simulink model "neptune_IDFT_HDL_Coder_input"  (R2023a)
settings: Solver=FixedStepDiscrete  StartTime=0.0  StopTime=20*(1/20000)  RelTol=1e-3  EnableMultiTasking=on
values from neighbouring files (symbols this model uses):
  AgcBurst = fi(AgcBurst)    [ofdm.m]
  PTT = timeseries(PTT, 1/22120448)    [ofdm.m]
undefined symbols (not defined in the file or in its folder): PreambleAlong, PreambleAshort, PreambleB
libraries: hdlsllib x10, dspsigops x4, commrandsrc3 x2, dsphdlxfrm2 x2, dspstat3 x1
settings Model: Creator=abraxas3d  LastModifiedBy=matt
settings OptimizationCC: BlockReduction=off  ConditionallyExecuteInputs=off  DefaultParameterBehavior=Inlined
settings DebuggingCC: AlgebraicLoopMsg=error  SingleTaskRateTransMsg=error
settings HardwareCC: ProdBitPerPointer=32  ProdBitPerSizeT=32  ProdBitPerPtrDiffT=32  ProdLargestAtomicFloat=None  ProdIntDivRoundTo=Undefined  ProdEndianess=Unspecified  ProdWordSize=32  ProdHWDeviceType=ASIC/FPGA->ASIC/FPGA  TargetBitPerLong=64  TargetBitPerPointer=64  TargetBitPerSizeT=64  TargetBitPerPtrDiffT=64  TargetLongLongMode=on  TargetIntDivRoundTo=Zero  TargetEndianess=LittleEndian  TargetWordSize=64  TargetHWDeviceType=Custom Processor->MATLAB Host Computer  ProdEqTarget=off

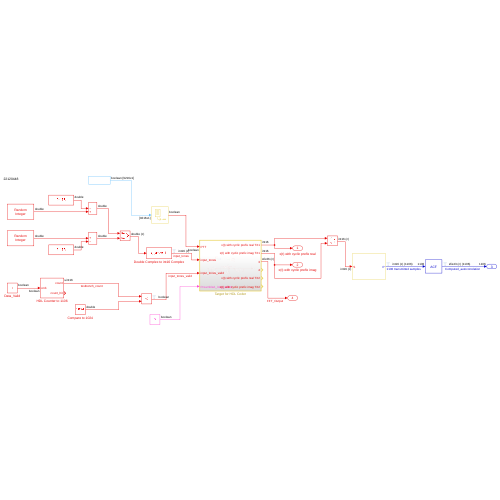
[thumbnail: Simulink's stored preview of the top-level diagram]
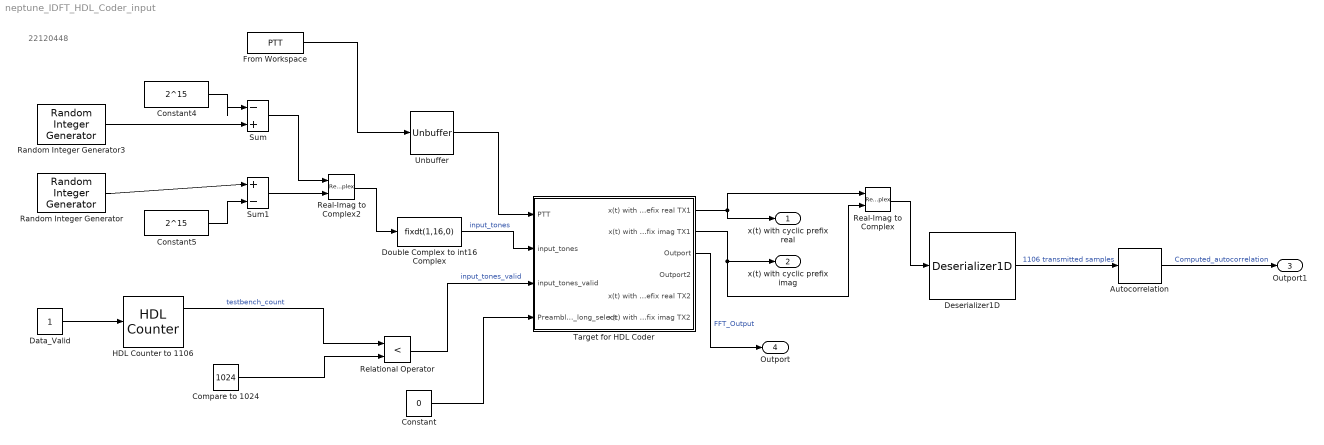
== system neptune_IDFT_HDL_Coder_input ==
  note: 22120448
  Autocorrelation : dspstat3/Autocorrelation  AllPositiveLags=on  maxlag=1105  bias=Unbiased  domain=Time  roundingMode=Floor  overflowMode=off  outputDataTypeStr=Inherit: Same as accumulator  outputMin=[]  outputMax=[]  outputLastDataTypeStr=Inherit: Same as accumulator
  Compare to 1024 : Constant  Value=1024  SampleTime=(1/22120448)
  Constant : Constant  Value=0  OutDataTypeStr=boolean
  Constant4 : Constant  Value=2^15  SampleTime=1/22120448
  Constant5 : Constant  Value=2^15  SampleTime=1/22120448
  Data_Valid : Constant  OutDataTypeStr=boolean  SampleTime=(1/22120448)
  Deserializer1D : hdlsllib/HDL Operations/Deserializer1D  Ratio=1106  IdleCycles=0  InitialCondition=0  startIn=off  validIn=off  validOut=off  inputDataDimensions=-1  inputSampleTime=-1  inputSignalType=complex
  Double Complex to int16 Complex : DataTypeConversion  OutMin=[-32768]  OutMax=[32767]  OutDataTypeStr=fixdt(1,16,0)  RndMeth=Floor
  From Workspace : FromWorkspace  VariableName=PTT  SampleTime=size(PTT.Data, 1)/22120448
  HDL Counter to 1106 : hdlsllib/Sources/HDL Counter  CountType=Count limited  CountInit=0  CountStep=1  CountMax=1105  CountFromType=Initial value  CountFrom=0  CountResetPort=off  CountLoadPort=off  CountEnbPort=on  CountDirPort=off  CountHitOutputPort=on  CountDataType=Unsigned  CountWordLen=16  CountFracLen=0  CountSampTime=1
  Random Integer Generator : commrandsrc3/Random Integer Generator  SetSize=2^16  SeedSource=Auto  Seed=0  SampleTime=1/22120448  SamplesPerFrame=1  OutputDataType=double  SimulateUsing=Interpreted execution
  Random Integer Generator3 : commrandsrc3/Random Integer Generator  SetSize=2^16  SeedSource=Auto  Seed=0  SampleTime=1/22120448  SamplesPerFrame=1  OutputDataType=double  SimulateUsing=Interpreted execution
  Real-Imag to Complex : RealImagToComplex
  Real-Imag to Complex2 : RealImagToComplex
  Relational Operator : RelationalOperator  Operator=<  OutDataTypeStr=boolean  InputSameDT=off
  Sum : Sum  Inputs=|-+
  Sum1 : Sum  Inputs=|+-
  Target for HDL Coder : Subsystem  TreatAsAtomicUnit=on
  Unbuffer : Unbuffer
  x(t) with cyclic prefix real : Outport
  x(t) with cyclic prefix imag : Outport  Port=2  VectorParamsAs1DForOutWhenUnconnected=off
  Outport1 : Outport  Port=3
  Outport : Outport  Port=4
  wires:
  Double Complex to int16 Complex/1 -> Target for HDL Coder/2(input_tones)  "input_tones"
  Target for HDL Coder/1(x(t) with cyclic prefix real TX1) -> x(t) with cyclic prefix real/1, Real-Imag to Complex/1
  Target for HDL Coder/2(x(t) with cyclic prefix imag TX1) -> Real-Imag to Complex/2, x(t) with cyclic prefix imag/1
  Compare to 1024/1 -> Relational Operator/2
  HDL Counter to 1106/1 -> Relational Operator/1  "testbench_count"
  Relational Operator/1 -> Target for HDL Coder/3(input_tones_valid)  "input_tones_valid"
  Data_Valid/1 -> HDL Counter to 1106/1
  Real-Imag to Complex/1 -> Deserializer1D/1
  Deserializer1D/1 -> Autocorrelation/1  "1106 transmitted samples"
  Autocorrelation/1 -> Outport1/1  "Computed_autocorrelation"
  Real-Imag to Complex2/1 -> Double Complex to int16 Complex/1
  Random Integer Generator3/1 -> Sum/2
  Constant4/1 -> Sum/1
  Sum/1 -> Real-Imag to Complex2/1
  Constant5/1 -> Sum1/2
  Random Integer Generator/1 -> Sum1/1
  Sum1/1 -> Real-Imag to Complex2/2
  Target for HDL Coder/3(Outport) -> Outport/1  "FFT_Output"
  Unbuffer/1 -> Target for HDL Coder/1(PTT)
  From Workspace/1 -> Unbuffer/1
  Constant/1 -> Target for HDL Coder/4(PreambleA_long_select)

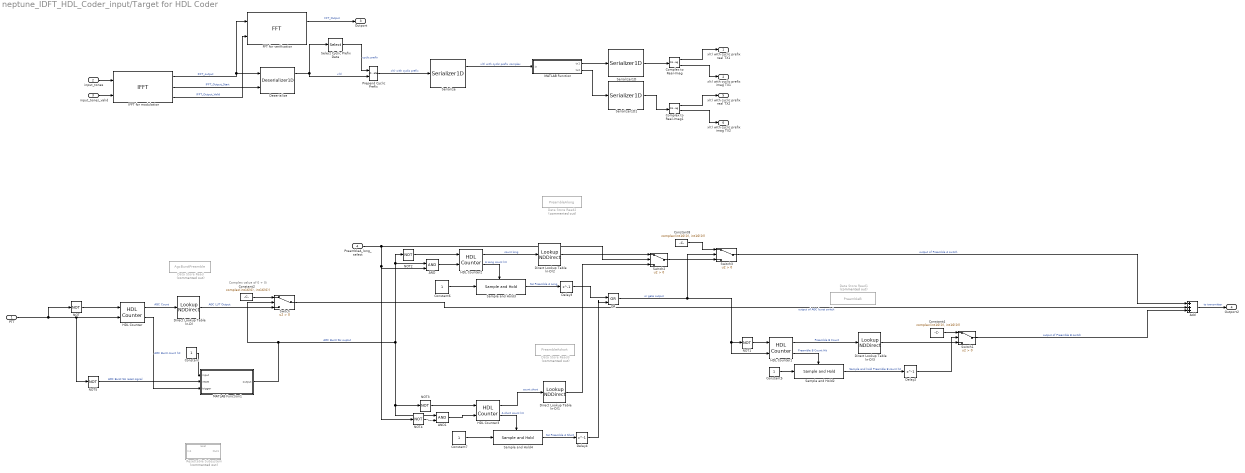
== system neptune_IDFT_HDL_Coder_input/Target for HDL Coder ==
  note: Complex value of 0 + 0i
  PTT : Inport  OutDataTypeStr=boolean
  input_tones : Inport  Port=2
  input_tones_valid : Inport  Port=3
  PreambleA_long_select : Inport  Port=4
  AND : Logic  IconShape=distinctive  AllPortsSameDT=off  OutDataTypeStr=boolean
  AND1 : Logic  IconShape=distinctive  AllPortsSameDT=off  OutDataTypeStr=boolean
  Add : Sum  Inputs=+++  OutDataTypeStr=fixdt(1,16,0)  SaturateOnIntegerOverflow=on
  Complex to Real-Imag : ComplexToRealImag
  Complex to Real-Imag1 : ComplexToRealImag
  Constant : Constant  OutDataTypeStr=boolean
  Constant2 : Constant  Value=complex(int16(0), int16(0))  VectorParams1D=off  OutDataTypeStr=int16
  Constant4 : Constant  Value=complex(int16(0), int16(0))  VectorParams1D=off  OutDataTypeStr=int16
  Constant5 : Constant  VectorParams1D=off  OutDataTypeStr=boolean  SampleTime=-1
  Constant6 : Constant  VectorParams1D=off  OutDataTypeStr=boolean  SampleTime=-1
  Constant7 : Constant  VectorParams1D=off  OutDataTypeStr=boolean  SampleTime=-1
  Constant8 : Constant  Value=complex(int16(0), int16(0))  VectorParams1D=off  OutDataTypeStr=int16
  Data Store Read : DataStoreRead  Commented=on  DataStoreName=AgcBurstPreamble  DataStoreElements=AgcBurstPreamble  EnableIndexing=on  IndexOptions=Index vector (port)  Indices=1  OutputSizes=1
  Data Store Read1 : DataStoreRead  Commented=on  DataStoreName=PreambleB  DataStoreElements=PreambleB  EnableIndexing=on  IndexOptions=Index vector (port)  Indices=1  OutputSizes=1
  Data Store Read2 : DataStoreRead  Commented=on  DataStoreName=PreambleAlong  DataStoreElements=PreambleAlong  EnableIndexing=on  IndexOptions=Index vector (port)  Indices=1  OutputSizes=1
  Data Store Read3 : DataStoreRead  Commented=on  DataStoreName=PreambleAshort  DataStoreElements=PreambleAshort  EnableIndexing=on  IndexOptions=Index vector (port)  Indices=1  OutputSizes=1
  Delay2 : Delay  DelayLength=1
  Delay3 : Delay  DelayLength=1
  Delay4 : Delay  DelayLength=1
  Deserialize : hdlsllib/HDL Operations/Deserializer1D  Ratio=1024  IdleCycles=82  InitialCondition=0  startIn=on  validIn=off  validOut=on  inputDataDimensions=-1  inputSampleTime=-1  inputSignalType=auto
  Direct Lookup Table (n-D) : LookupNDDirect  NumberOfTableDimensions=1  Table=AgcBurst  DiagnosticForOutOfRangeInput=Error
  Direct Lookup Table (n-D)1 : LookupNDDirect  NumberOfTableDimensions=1  Table=PreambleAshort  DiagnosticForOutOfRangeInput=Error
  Direct Lookup Table (n-D)2 : LookupNDDirect  NumberOfTableDimensions=1  Table=PreambleAlong  DiagnosticForOutOfRangeInput=Error
  Direct Lookup Table (n-D)3 : LookupNDDirect  NumberOfTableDimensions=1  Table=PreambleB  DiagnosticForOutOfRangeInput=Error
  FFT for verification : dsphdlxfrm2/FFT  FFTLength=1024  Architecture=Streaming Radix 2^2  ComplexMultiplication=Use 4 multipliers and 2 adders  BitReversedOutput=off  BitReversedInput=on  Normalize=off  SimulateUsing=Code generation  RoundingMethod=Floor  ResetInputPort=off  StartOutputPort=off  EndOutputPort=off
  HDL Counter : hdlsllib/Sources/HDL Counter  CountType=Count limited  CountInit=0  CountStep=1  CountMax=109  CountFromType=Initial value  CountFrom=0  CountResetPort=on  CountLoadPort=off  CountEnbPort=on  CountDirPort=off  CountHitOutputPort=on  CountDataType=Unsigned  CountWordLen=8  CountFracLen=0  CountSampTime=1
  HDL Counter1 : hdlsllib/Sources/HDL Counter  CountType=Count limited  CountInit=0  CountStep=1  CountMax=1024  CountFromType=Initial value  CountFrom=0  CountResetPort=on  CountLoadPort=off  CountEnbPort=on  CountDirPort=off  CountHitOutputPort=on  CountDataType=Unsigned  CountWordLen=16  CountFracLen=0  CountSampTime=1
  HDL Counter2 : hdlsllib/Sources/HDL Counter  CountType=Count limited  CountInit=1  CountStep=1  CountMax=5530  CountFromType=Initial value  CountFrom=1  CountResetPort=on  CountLoadPort=off  CountEnbPort=on  CountDirPort=off  CountHitOutputPort=on  CountDataType=Unsigned  CountWordLen=16  CountFracLen=0  CountSampTime=1
  HDL Counter3 : hdlsllib/Sources/HDL Counter  CountType=Count limited  CountInit=0  CountStep=1  CountMax=552  CountFromType=Initial value  CountFrom=0  CountResetPort=on  CountLoadPort=off  CountEnbPort=on  CountDirPort=off  CountHitOutputPort=on  CountDataType=Unsigned  CountWordLen=16  CountFracLen=0  CountSampTime=1
  IFFT for modulation : dsphdlxfrm2/IFFT  FFTLength=IFFTsize  Architecture=Streaming Radix 2^2  ComplexMultiplication=Use 4 multipliers and 2 adders  BitReversedOutput=on  BitReversedInput=off  Normalize=on  SimulateUsing=Code generation  RoundingMethod=Floor  ResetInputPort=off  StartOutputPort=on  EndOutputPort=off
  MATLAB Function : MATLAB Function  TreatAsAtomicUnit=on
  MATLAB Function1 : MATLAB Function  TreatAsAtomicUnit=on
  NOT{,1..5} (6 alike) : Logic  Operator=NOT  IconShape=distinctive  AllPortsSameDT=off  OutDataTypeStr=boolean
  OR : Logic  Operator=OR  IconShape=distinctive  AllPortsSameDT=off  OutDataTypeStr=boolean
  Prepend Cyclic Prefix : Concatenate
  Resettable Subsystem : Subsystem  Commented=on  TreatAsAtomicUnit=on
  Sample and Hold2 : dspsigops/Sample and Hold  trig=Rising edge  initCond=0  latchinput=off
  Sample and Hold3 : dspsigops/Sample and Hold  trig=Rising edge  initCond=0  latchinput=off
  Sample and Hold4 : dspsigops/Sample and Hold  trig=Rising edge  initCond=0  latchinput=off
  Select Cyclic Prefix Data : Selector  InputPortWidth=1024  IndexOptions=Index vector (dialog)  Indices=[1024-81:1024]  OutputSizes=1
  Serialize : hdlsllib/HDL Operations/Serializer1D  Ratio=1106/2  IdleCycles=0  validIn=off  startOut=off  validOut=on  inputDataDimensions=-1  inputSampleTime=-1  inputSignalType=auto
  Serializer1D : hdlsllib/HDL Operations/Serializer1D  Ratio=2  IdleCycles=0  validIn=off  startOut=off  validOut=off  inputDataDimensions=-1  inputSampleTime=-1  inputSignalType=auto
  Serializer1D1 : hdlsllib/HDL Operations/Serializer1D  Ratio=2  IdleCycles=0  validIn=off  startOut=off  validOut=off  inputDataDimensions=-1  inputSampleTime=-1  inputSignalType=auto
  Switch{,1..3} (4 alike) : Switch  Criteria=u2 > Threshold  SaturateOnIntegerOverflow=off  InputSameDT=off
  x(t) with cyclic prefix real TX1 : Outport  VectorParamsAs1DForOutWhenUnconnected=off
  x(t) with cyclic prefix imag TX1 : Outport  Port=2  VectorParamsAs1DForOutWhenUnconnected=off
  Outport : Outport  Port=3
  Outport2 : Outport  Port=4
  x(t) with cyclic prefix real TX2 : Outport  Port=5  VectorParamsAs1DForOutWhenUnconnected=off
  x(t) with cyclic prefix imag TX2 : Outport  Port=6  VectorParamsAs1DForOutWhenUnconnected=off
  wires:
  Deserialize/1 -> Select Cyclic Prefix Data/1, Prepend Cyclic Prefix/2  "x(t)"
  Select Cyclic Prefix Data/1 -> Prepend Cyclic Prefix/1  "cyclic prefix"
  input_tones_valid/1 -> IFFT for modulation/2
  IFFT for modulation/1 -> FFT for verification/1, Deserialize/1  "IFFT_output"
  Prepend Cyclic Prefix/1 -> Serialize/1  "x(t) with cyclic prefix"
  Complex to Real-Imag/2 -> x(t) with cyclic prefix imag TX1/1
  Complex to Real-Imag/1 -> x(t) with cyclic prefix real TX1/1
  Serialize/1 -> MATLAB Function/1(in)  "x(t) with cyclic prefix complex"
  IFFT for modulation/2 -> Deserialize/2  "IFFT_Output_Start"
  FFT for verification/1 -> Outport/1  "FFT_Output"
  input_tones/1 -> IFFT for modulation/1
  IFFT for modulation/3 -> FFT for verification/2  "IFFT_Output_Valid"
  PTT/1 -> NOT/1, NOT5/1, HDL Counter/2
  HDL Counter/1 -> Direct Lookup Table (n-D)/1  "AGC Count"
  NOT/1 -> HDL Counter/1
  Constant2/1 -> Switch/1
  OR/1 -> Switch3/2, HDL Counter1/2, NOT1/1  "or gate output"
  NOT1/1 -> HDL Counter1/1
  Constant4/1 -> Switch1/1
  HDL Counter1/1 -> Direct Lookup Table (n-D)3/1  "Preamble B Count"
  Switch/1 -> Add/2  "output of AGC burst switch"
  Switch1/1 -> Add/3  "output of Preamble B switch"
  Add/1 -> Outport2/1  "to transmitter"
  PreambleA_long_select/1 -> NOT4/1, AND/2, Switch2/2
  Constant5/1 -> Sample and Hold2/1
  HDL Counter1/2 -> Sample and Hold2/Trigger  "Preamble B Count Hit"
  Sample and Hold2/1 -> Delay2/1  "Sample and hold Preamble B count hit"
  NOT2/1 -> HDL Counter2/1
  HDL Counter2/1 -> Direct Lookup Table (n-D)2/1  "count long"
  Constant6/1 -> Sample and Hold3/1
  HDL Counter2/2 -> Sample and Hold3/Trigger  "A Long count hit"
  Sample and Hold3/1 -> Delay3/1  "SH Preamble A Long"
  NOT3/1 -> HDL Counter3/1
  Constant7/1 -> Sample and Hold4/1
  HDL Counter3/2 -> Sample and Hold4/Trigger  "A short count hit"
  Sample and Hold4/1 -> Delay4/1  "SH Preamble A Short"
  Delay3/1 -> OR/1
  Delay4/1 -> OR/2
  HDL Counter3/1 -> Direct Lookup Table (n-D)1/1  "count short"
  Switch3/1 -> Add/1  "output of Preamble A switch"
  Constant8/1 -> Switch3/1
  Switch2/1 -> Switch3/3
  AND/1 -> HDL Counter2/2
  AND1/1 -> HDL Counter3/2
  NOT4/1 -> AND1/2
  Delay2/1 -> Switch1/2
  HDL Counter/2 -> MATLAB Function1/3(trigger)  "AGC Burst count hit"
  MATLAB Function1/1(output) -> Switch/2, NOT3/1, AND1/1, NOT2/1, AND/1  "AGC Burst SH ouptut"
  NOT5/1 -> MATLAB Function1/2(reset)  "AGC Burst SH reset signal"
  MATLAB Function/1(tx1) -> Serializer1D/1
  Serializer1D/1 -> Complex to Real-Imag/1
  MATLAB Function/2(tx2) -> Serializer1D1/1
  Serializer1D1/1 -> Complex to Real-Imag1/1
  Complex to Real-Imag1/1 -> x(t) with cyclic prefix real TX2/1
  Complex to Real-Imag1/2 -> x(t) with cyclic prefix imag TX2/1
  Direct Lookup Table (n-D)/1 -> Switch/3  "AGC LUT Output"
  Direct Lookup Table (n-D)2/1 -> Switch2/1
  Direct Lookup Table (n-D)1/1 -> Switch2/3
  Direct Lookup Table (n-D)3/1 -> Switch1/3
  Constant/1 -> MATLAB Function1/1(input)

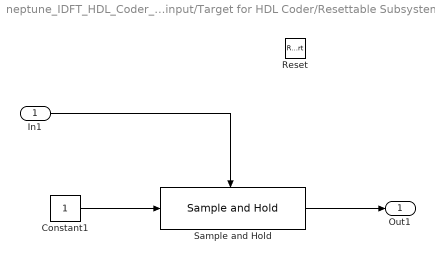
== system neptune_IDFT_HDL_Coder_input/Target for HDL Coder/Resettable Subsystem ==
  In1 : Inport
  Reset : ResetPort  DisableCoverage=on
  Constant1 : Constant  VectorParams1D=off  OutDataTypeStr=boolean  SampleTime=1/22120448
  Sample and Hold : dspsigops/Sample and Hold  trig=Rising edge  initCond=0  latchinput=off
  Out1 : Outport
  wires:
  Constant1/1 -> Sample and Hold/1
  In1/1 -> Sample and Hold/Trigger
  Sample and Hold/1 -> Out1/1

== matlab function neptune_IDFT_HDL_Coder_input/Target for HDL Coder/MATLAB Function ==
  settings: updateMethod=DISCRETE
  data: in input; tx1 output; tx2 output
function [tx1, tx2] = neptune_sfbc(in)
%Neptune space frequency block code
%   for two transmit antennas, space frequency block coding is implemented.
%   "in" is arriving as a 2 by 1 column vector. 
persistent hTDEnc;
if isempty(hTDEnc)
    %use same object for both STBC and SFBC - clever coding from 
    % "Understanding LTE with MATLAB" by Houman Zarinnkoub. 
    hTDEnc = comm.OSTBCEncoder('NumTransmitAntennas', 2);
end
new_imaginary = -1*imag(in(2));
new_real = -1*real(in(2));
neg_conj_in2 = complex(new_real, new_imaginary);

new_imaginary = -1*imag(in(1));
new_real = real(in(1));
conj_in1 = complex(new_real, new_imaginary);

tx1 = [in(1); in(2)];
tx2 = [neg_conj_in2; conj_in1];

end

== matlab function neptune_IDFT_HDL_Coder_input/Target for HDL Coder/MATLAB Function1 ==
  data: input input; output output; reset input; trigger input
function output   = resettable_sample_and_hold(input, reset, trigger)
%#codegen

%Resettable Sample and Hold Circuit
% This was written because S&H within Resettable Subsystems in Simulink
% is not supported by HDL Coder. We needed this functionality, so this
% custom function was written. 



initial_value = false;

    persistent sample_held;
    if isempty(sample_held)
        sample_held = false;
    end

    persistent output_held_value;
    if isempty(output_held_value)
        output_held_value = false;
    end


switch reset
    case 0 % not in reset
        %output = initial_value; % may not need this
        switch trigger
            case 0
                output = output_held_value;
            case 1
                if sample_held == false
                    output_held_value = input;
                    output = output_held_value;
                    sample_held = true;
                else
                    output = output_held_value;
                end
            otherwise
                output = initial_value;
        end
    case 1 % reset signal received
        output = initial_value;
        sample_held = false;
        output_held_value = false;
    otherwise
        output = initial_value;
        
end
